simulink model "BrowarModel"  (R2024a)
settings: Solver=ode5  StartTime=0.0  StopTime=inf  FixedStep=0.1  RelTol=1e-3
undefined symbols (not defined in the file or in its folder): localhost, Matrikon, OI
libraries: opclib x24
(part 3 of 9)

== system BrowarModel/Kadz zacierna/FT201 ==
  note: Przetwornik pomiarowy
  In : Inport
  F_gain : Gain  Gain=0
  F_offset : Constant  Value=0
  GUIMon : Gain
  Kompensacja : Constant  Value=Kompensacja
  Product : Product  RndMeth=Zero
  Saturation : Saturate  UpperLimit=100  LowerLimit=0
  Skalowanie (0-100%) : Gain  Gain=100/SrcZakres
  Sum{,1..3} (4 alike) : Sum  Inputs=|++
  Transfer Fcn : TransferFcn  Denominator=[0.3 1]
  Zaklocenia pomiarowe : Subsystem
  Zakres : Constant  Value=Zakres/100
  Out : Outport
  wires:
  Transfer Fcn/1 -> Saturation/1
  F_offset/1 -> Sum3/2
  F_gain/1 -> Sum2/2
  Product/1 -> Sum/1
  Zakres/1 -> Product/2
  Kompensacja/1 -> Sum/2
  Sum/1 -> GUIMon/1
  Skalowanie (0-100%)/1 -> Sum1/1
  Zaklocenia pomiarowe/1(Out) -> Sum1/2
  Sum1/1 -> F_gain/1, Sum2/1
  Sum3/1 -> Transfer Fcn/1
  Sum2/1 -> Sum3/1
  In/1 -> Skalowanie (0-100%)/1
  GUIMon/1 -> Out/1
  Saturation/1 -> Product/1

== system BrowarModel/Kadz zacierna/Kadz zacierna ==
  note: Kadz zacierna
  "Doplyw wody " : Inport
  Doplyw sruty : Inport  Port=2
  Zalaczenie silnika : Inport  Port=3
  "Zadane obroty silnika " : Inport  Port=4
  Sterowanie ogrzewaczem : Inport  Port=5
  Odplyw : Inport  Port=6
  F{211..214,221,231..232,241} (8 alike) : Constant  Value=0
  Kadz zacierna : Subsystem
  Model mieszadla : Subsystem
  Model ogrzewacza : Subsystem
  Silnik elektryczny : Subsystem
  Temperatura sruty : Constant  Value=22
  Temperatura wody : Constant  Value=22
  Terminator1 : Terminator
  Zawor doplywu wody : Subsystem  mask{Fmax=0.2}
      mask prompts: Fmax "Przeplyw maksymalny [m3/s]"
  Poziom : Outport
  Poziom wysoki : Outport  Port=2
  Poziom niski : Outport  Port=3
  Przeplyw wody : Outport  Port=4
  Sensor temperatury gorny : Outport  Port=5
  Sensor temperatury srodkowy : Outport  Port=6
  Sensor temperatury dolny : Outport  Port=7
  Obroty silnika : Outport  Port=8
  Prad silnika : Outport  Port=9
  Silnik Idle : Outport  Port=10
  Silnik Running : Outport  Port=11
  Silnik Alarm : Outport  Port=12
  Jakosc zacieru : Outport  Port=13
  Temperatura : Outport  Port=14
  wires:
  Model mieszadla/1(Obroty zredukowane) -> Kadz zacierna/7(Obroty mieszadla)
  Sterowanie ogrzewaczem/1 -> Model ogrzewacza/1(Sterowanie)
  Doplyw sruty/1 -> Kadz zacierna/3(Doplyw sruty)  "m3/h"
  Kadz zacierna/4(Temperatura sensor gorny) -> Sensor temperatury gorny/1
  Kadz zacierna/5(Temperatura sensor srodkowy) -> Sensor temperatury srodkowy/1
  Kadz zacierna/6(Temperatura sensor dolny) -> Sensor temperatury dolny/1
  Model ogrzewacza/1(Cieplo dostarczone) -> Kadz zacierna/6(Dostepny strumien ciepla)
  Kadz zacierna/1(Poziom) -> Poziom/1, Model mieszadla/1(Poziom)
  Kadz zacierna/2(Poziom wysoki) -> Poziom wysoki/1
  Kadz zacierna/3(Poziom niski) -> Poziom niski/1
  Odplyw/1 -> Kadz zacierna/5(Odplyw)  "m3/s"
  Temperatura wody/1 -> Kadz zacierna/2(Temperatura doplywu wody)
  Temperatura sruty/1 -> Kadz zacierna/4(Temperatura doplywu sruty)
  F221/1 -> Kadz zacierna/8(Wyciek)
  Zalaczenie silnika/1 -> Silnik elektryczny/1(Zalaczenie)
  "Zadane obroty silnika "/1 -> Silnik elektryczny/2(Zadane obroty)
  F232/1 -> Silnik elektryczny/4(Uszkodzenie)
  Model mieszadla/2(Obciazenie) -> Silnik elektryczny/3(Obciazenie zew)
  F231/1 -> Model mieszadla/3(Poslizg przekladni)
  Kadz zacierna/8(Jakosc zacieru) -> Jakosc zacieru/1
  F211/1 -> Zawor doplywu wody/2(Dlawienie)
  "Doplyw wody "/1 -> Zawor doplywu wody/1(Sterowanie)
  F212/1 -> Zawor doplywu wody/3(Przeciek)
  F213/1 -> Zawor doplywu wody/4(Wyciek)
  F214/1 -> Zawor doplywu wody/5(Brak)
  Zawor doplywu wody/1(Przeplyw) -> Przeplyw wody/1, Kadz zacierna/1(Doplyw wody)
  Silnik elektryczny/1(Obroty) -> Model mieszadla/2(Obroty), Obroty silnika/1
  Silnik elektryczny/2(Prad) -> Prad silnika/1
  Silnik elektryczny/3(Idle) -> Silnik Idle/1
  Silnik elektryczny/4(Running) -> Silnik Running/1
  Silnik elektryczny/5(Alarm) -> Silnik Alarm/1
  Kadz zacierna/7(Temperatura dna) -> Terminator1/1
  F241/1 -> Model ogrzewacza/2(Spadek mocy)
  Kadz zacierna/9(Temperatura srednia) -> Temperatura/1

== system BrowarModel/Kadz zacierna/LT202 ==
  note: Przetwornik pomiarowy
  In : Inport
  F_gain : Gain  Gain=0
  F_offset : Constant  Value=0
  GUIMon : Gain
  Kompensacja : Constant  Value=Kompensacja
  Product : Product  RndMeth=Zero
  Saturation : Saturate  UpperLimit=100  LowerLimit=0
  Skalowanie (0-100%) : Gain  Gain=100/SrcZakres
  Sum{,1..3} (4 alike) : Sum  Inputs=|++
  Transfer Fcn : TransferFcn  Denominator=[0.3 1]
  Zaklocenia pomiarowe : Subsystem
  Zakres : Constant  Value=Zakres/100
  Out : Outport
  wires:
  Saturation/1 -> Product/1
  GUIMon/1 -> Out/1
  In/1 -> Skalowanie (0-100%)/1
  Sum2/1 -> Sum3/1
  Sum3/1 -> Transfer Fcn/1
  Sum1/1 -> Sum2/1, F_gain/1
  Zaklocenia pomiarowe/1(Out) -> Sum1/2
  Skalowanie (0-100%)/1 -> Sum1/1
  Sum/1 -> GUIMon/1
  Kompensacja/1 -> Sum/2
  Zakres/1 -> Product/2
  Product/1 -> Sum/1
  F_gain/1 -> Sum2/2
  F_offset/1 -> Sum3/2
  Transfer Fcn/1 -> Saturation/1

== system BrowarModel/Kadz zacierna/LT202H ==
  note: Przetwornik pomiarowy
  In : Inport
  FT : Constant  Value=0
  FT_value : Constant  Value=0
  GUIMon : Gain
  Switch : Switch  Threshold=0.5  SaturateOnIntegerOverflow=off  InputSameDT=off
  Out : Outport
  wires:
  In/1 -> Switch/3
  GUIMon/1 -> Out/1
  FT/1 -> Switch/2
  Switch/1 -> GUIMon/1
  FT_value/1 -> Switch/1

== system BrowarModel/Kadz zacierna/LT202L ==
  note: Przetwornik pomiarowy
  In : Inport
  FT : Constant  Value=0
  FT_value : Constant  Value=0
  GUIMon : Gain
  Switch : Switch  Threshold=0.5  SaturateOnIntegerOverflow=off  InputSameDT=off
  Out : Outport
  wires:
  FT_value/1 -> Switch/1
  Switch/1 -> GUIMon/1
  FT/1 -> Switch/2
  GUIMon/1 -> Out/1
  In/1 -> Switch/3

== system BrowarModel/Kadz zacierna/LV201 ==
  note: Sterowanie
  GUIMon : Gain
  Lokalne : Constant  Value=0
  Wybor : Switch  Threshold=0.5  SaturateOnIntegerOverflow=off  InputSameDT=off
  Out : Outport
  wires:
  GUIMon/1 -> Out/1
  Wybor/1 -> GUIMon/1
  [TrybSter] -> Wybor/2
  [LV201] -> Wybor/1
  Lokalne/1 -> Wybor/3

== system BrowarModel/Kadz zacierna/QT204 ==
  note: Przetwornik pomiarowy
  In : Inport
  FT : Constant  Value=0
  FT_value : Constant  Value=0
  GUIMon : Gain
  Granica : Constant  Value=0.8
  Saturation : Saturate  UpperLimit=1  LowerLimit=0
  Saturation1 : Saturate  UpperLimit=1  LowerLimit=0
  Sensor max : RelationalOperator  InputSameDT=off
  Sum5 : Sum  Inputs=|++
  Switch : Switch  Threshold=0.5  SaturateOnIntegerOverflow=off  InputSameDT=off
  Zaklocenia : Subsystem
  Out : Outport
  wires:
  FT_value/1 -> Switch/1
  Switch/1 -> GUIMon/1
  FT/1 -> Switch/2
  GUIMon/1 -> Out/1
  In/1 -> Saturation/1
  Saturation1/1 -> Switch/3
  Saturation/1 -> Sum5/1, Zaklocenia/1(In)
  Sum5/1 -> Sensor max/1
  Zaklocenia/1(Out) -> Sum5/2
  Granica/1 -> Sensor max/2
  Sensor max/1 -> Saturation1/1

== system BrowarModel/Kadz zacierna/ST205 ==
  note: Przetwornik pomiarowy
  In : Inport
  F_gain : Gain  Gain=0
  F_offset : Constant  Value=0
  GUIMon : Gain
  Kompensacja : Constant  Value=Kompensacja
  Product : Product  RndMeth=Zero
  Saturation : Saturate  UpperLimit=100  LowerLimit=0
  Skalowanie (0-100%) : Gain  Gain=100/SrcZakres
  Sum{,1..3} (4 alike) : Sum  Inputs=|++
  Transfer Fcn : TransferFcn  Denominator=[0.3 1]
  Zaklocenia pomiarowe : Subsystem
  Zakres : Constant  Value=Zakres/100
  Out : Outport
  wires:
  Saturation/1 -> Product/1
  GUIMon/1 -> Out/1
  In/1 -> Skalowanie (0-100%)/1
  Sum2/1 -> Sum3/1
  Sum3/1 -> Transfer Fcn/1
  Sum1/1 -> Sum2/1, F_gain/1
  Zaklocenia pomiarowe/1(Out) -> Sum1/2
  Skalowanie (0-100%)/1 -> Sum1/1
  Sum/1 -> GUIMon/1
  Kompensacja/1 -> Sum/2
  Zakres/1 -> Product/2
  Product/1 -> Sum/1
  F_gain/1 -> Sum2/2
  F_offset/1 -> Sum3/2
  Transfer Fcn/1 -> Saturation/1

== system BrowarModel/Kadz zacierna/TT203H ==
  note: Przetwornik pomiarowy
  In : Inport
  F_gain : Gain  Gain=0
  F_offset : Constant  Value=0
  GUIMon : Gain
  Kompensacja : Constant  Value=Kompensacja
  Product : Product  RndMeth=Zero
  Saturation : Saturate  UpperLimit=100  LowerLimit=0
  Skalowanie (0-100%) : Gain  Gain=100/SrcZakres
  Sum{,1..3} (4 alike) : Sum  Inputs=|++
  Transfer Fcn : TransferFcn  Denominator=[0.3 1]
  Zaklocenia pomiarowe : Subsystem
  Zakres : Constant  Value=Zakres/100
  Out : Outport
  wires:
  Transfer Fcn/1 -> Saturation/1
  F_offset/1 -> Sum3/2
  F_gain/1 -> Sum2/2
  Product/1 -> Sum/1
  Zakres/1 -> Product/2
  Kompensacja/1 -> Sum/2
  Sum/1 -> GUIMon/1
  Skalowanie (0-100%)/1 -> Sum1/1
  Zaklocenia pomiarowe/1(Out) -> Sum1/2
  Sum1/1 -> F_gain/1, Sum2/1
  Sum3/1 -> Transfer Fcn/1
  Sum2/1 -> Sum3/1
  In/1 -> Skalowanie (0-100%)/1
  GUIMon/1 -> Out/1
  Saturation/1 -> Product/1

== system BrowarModel/Kadz zacierna/TT203L ==
  note: Przetwornik pomiarowy
  In : Inport
  F_gain : Gain  Gain=0
  F_offset : Constant  Value=0
  GUIMon : Gain
  Kompensacja : Constant  Value=Kompensacja
  Product : Product  RndMeth=Zero
  Saturation : Saturate  UpperLimit=100  LowerLimit=0
  Skalowanie (0-100%) : Gain  Gain=100/SrcZakres
  Sum{,1..3} (4 alike) : Sum  Inputs=|++
  Transfer Fcn : TransferFcn  Denominator=[0.3 1]
  Zaklocenia pomiarowe : Subsystem
  Zakres : Constant  Value=Zakres/100
  Out : Outport
  wires:
  Transfer Fcn/1 -> Saturation/1
  F_offset/1 -> Sum3/2
  F_gain/1 -> Sum2/2
  Product/1 -> Sum/1
  Zakres/1 -> Product/2
  Kompensacja/1 -> Sum/2
  Sum/1 -> GUIMon/1
  Skalowanie (0-100%)/1 -> Sum1/1
  Zaklocenia pomiarowe/1(Out) -> Sum1/2
  Sum1/1 -> F_gain/1, Sum2/1
  Sum3/1 -> Transfer Fcn/1
  Sum2/1 -> Sum3/1
  In/1 -> Skalowanie (0-100%)/1
  GUIMon/1 -> Out/1
  Saturation/1 -> Product/1

== system BrowarModel/Kadz zacierna/TT203M ==
  note: Przetwornik pomiarowy
  In : Inport
  F_gain : Gain  Gain=0
  F_offset : Constant  Value=0
  GUIMon : Gain
  Kompensacja : Constant  Value=Kompensacja
  Product : Product  RndMeth=Zero
  Saturation : Saturate  UpperLimit=100  LowerLimit=0
  Skalowanie (0-100%) : Gain  Gain=100/SrcZakres
  Sum{,1..3} (4 alike) : Sum  Inputs=|++
  Transfer Fcn : TransferFcn  Denominator=[0.3 1]
  Zaklocenia pomiarowe : Subsystem
  Zakres : Constant  Value=Zakres/100
  Out : Outport
  wires:
  Saturation/1 -> Product/1
  GUIMon/1 -> Out/1
  In/1 -> Skalowanie (0-100%)/1
  Sum2/1 -> Sum3/1
  Sum3/1 -> Transfer Fcn/1
  Sum1/1 -> Sum2/1, F_gain/1
  Zaklocenia pomiarowe/1(Out) -> Sum1/2
  Skalowanie (0-100%)/1 -> Sum1/1
  Sum/1 -> GUIMon/1
  Kompensacja/1 -> Sum/2
  Zakres/1 -> Product/2
  Product/1 -> Sum/1
  F_gain/1 -> Sum2/2
  F_offset/1 -> Sum3/2
  Transfer Fcn/1 -> Saturation/1

== system BrowarModel/Kadz zacierna/TV203 ==
  note: Sterowanie
  GUIMon : Gain
  Lokalne : Constant  Value=0
  Wybor : Switch  Threshold=0.5  SaturateOnIntegerOverflow=off  InputSameDT=off
  Out : Outport
  wires:
  Lokalne/1 -> Wybor/3
  [TV203] -> Wybor/1
  [TrybSter] -> Wybor/2
  Wybor/1 -> GUIMon/1
  GUIMon/1 -> Out/1

== system BrowarModel/Kadz zacierna/XV205 ==
  note: Sterowanie
  GUIMon : Gain
  Lokalne : Constant  Value=0
  Wybor : Switch  Threshold=0.5  SaturateOnIntegerOverflow=off  InputSameDT=off
  Out : Outport
  wires:
  Lokalne/1 -> Wybor/3
  [XV205] -> Wybor/1
  [TrybSter] -> Wybor/2
  Wybor/1 -> GUIMon/1
  GUIMon/1 -> Out/1

== system BrowarModel/Kadz zacierna/XV205SP ==
  note: Sterowanie
  GUIMon : Gain
  Lokalne : Constant  Value=100
  Wybor : Switch  Threshold=0.5  SaturateOnIntegerOverflow=off  InputSameDT=off
  Out : Outport
  wires:
  Lokalne/1 -> Wybor/3
  [XV205SP] -> Wybor/1
  [TrybSter] -> Wybor/2
  Wybor/1 -> GUIMon/1
  GUIMon/1 -> Out/1

== system BrowarModel/Mlyn browarniany/ET103 ==
  note: Przetwornik pomiarowy
  In : Inport
  F_gain : Gain  Gain=0
  F_offset : Constant  Value=0
  GUIMon : Gain
  Kompensacja : Constant  Value=Kompensacja
  Product : Product  RndMeth=Zero
  Saturation : Saturate  UpperLimit=100  LowerLimit=0
  Skalowanie (0-100%) : Gain  Gain=100/SrcZakres
  Sum{,1..3} (4 alike) : Sum  Inputs=|++
  Transfer Fcn : TransferFcn  Denominator=[0.3 1]
  Zaklocenia pomiarowe : Subsystem
  Zakres : Constant  Value=Zakres/100
  Out : Outport
  wires:
  Transfer Fcn/1 -> Saturation/1
  F_offset/1 -> Sum3/2
  F_gain/1 -> Sum2/2
  Product/1 -> Sum/1
  Zakres/1 -> Product/2
  Kompensacja/1 -> Sum/2
  Sum/1 -> GUIMon/1
  Skalowanie (0-100%)/1 -> Sum1/1
  Zaklocenia pomiarowe/1(Out) -> Sum1/2
  Sum1/1 -> F_gain/1, Sum2/1
  Sum3/1 -> Transfer Fcn/1
  Sum2/1 -> Sum3/1
  In/1 -> Skalowanie (0-100%)/1
  GUIMon/1 -> Out/1
  Saturation/1 -> Product/1

== system BrowarModel/Mlyn browarniany/ET105 ==
  note: Przetwornik pomiarowy
  In : Inport
  F_gain : Gain  Gain=0
  F_offset : Constant  Value=0
  GUIMon : Gain
  Kompensacja : Constant  Value=Kompensacja
  Product : Product  RndMeth=Zero
  Saturation : Saturate  UpperLimit=100  LowerLimit=0
  Skalowanie (0-100%) : Gain  Gain=100/SrcZakres
  Sum{,1..3} (4 alike) : Sum  Inputs=|++
  Transfer Fcn : TransferFcn  Denominator=[0.3 1]
  Zaklocenia pomiarowe : Subsystem
  Zakres : Constant  Value=Zakres/100
  Out : Outport
  wires:
  Saturation/1 -> Product/1
  GUIMon/1 -> Out/1
  In/1 -> Skalowanie (0-100%)/1
  Sum2/1 -> Sum3/1
  Sum3/1 -> Transfer Fcn/1
  Sum1/1 -> Sum2/1, F_gain/1
  Zaklocenia pomiarowe/1(Out) -> Sum1/2
  Skalowanie (0-100%)/1 -> Sum1/1
  Sum/1 -> GUIMon/1
  Kompensacja/1 -> Sum/2
  Zakres/1 -> Product/2
  Product/1 -> Sum/1
  F_gain/1 -> Sum2/2
  F_offset/1 -> Sum3/2
  Transfer Fcn/1 -> Saturation/1

== system BrowarModel/Mlyn browarniany/FT105 ==
  note: Przetwornik pomiarowy
  In : Inport
  F_gain : Gain  Gain=0
  F_offset : Constant  Value=0
  GUIMon : Gain
  Kompensacja : Constant  Value=Kompensacja
  Product : Product  RndMeth=Zero
  Saturation : Saturate  UpperLimit=100  LowerLimit=0
  Skalowanie (0-100%) : Gain  Gain=100/SrcZakres
  Sum{,1..3} (4 alike) : Sum  Inputs=|++
  Transfer Fcn : TransferFcn  Denominator=[0.3 1]
  Zaklocenia pomiarowe : Subsystem
  Zakres : Constant  Value=Zakres/100
  Out : Outport
  wires:
  Saturation/1 -> Product/1
  GUIMon/1 -> Out/1
  In/1 -> Skalowanie (0-100%)/1
  Sum2/1 -> Sum3/1
  Sum3/1 -> Transfer Fcn/1
  Sum1/1 -> Sum2/1, F_gain/1
  Zaklocenia pomiarowe/1(Out) -> Sum1/2
  Skalowanie (0-100%)/1 -> Sum1/1
  Sum/1 -> GUIMon/1
  Kompensacja/1 -> Sum/2
  Zakres/1 -> Product/2
  Product/1 -> Sum/1
  F_gain/1 -> Sum2/2
  F_offset/1 -> Sum3/2
  Transfer Fcn/1 -> Saturation/1

== system BrowarModel/Mlyn browarniany/FV103 ==
  note: Sterowanie
  GUIMon : Gain
  Lokalne : Constant  Value=0
  Wybor : Switch  Threshold=0.5  SaturateOnIntegerOverflow=off  InputSameDT=off
  Out : Outport
  wires:
  Lokalne/1 -> Wybor/3
  [FV103] -> Wybor/1
  [TrybSter] -> Wybor/2
  Wybor/1 -> GUIMon/1
  GUIMon/1 -> Out/1

== system BrowarModel/Mlyn browarniany/FV103SP ==
  note: Sterowanie
  GUIMon : Gain
  Lokalne : Constant  Value=65.3333
  Wybor : Switch  Threshold=0.5  SaturateOnIntegerOverflow=off  InputSameDT=off
  Out : Outport
  wires:
  GUIMon/1 -> Out/1
  Wybor/1 -> GUIMon/1
  [TrybSter] -> Wybor/2
  [FV103SP] -> Wybor/1
  Lokalne/1 -> Wybor/3

== system BrowarModel/Mlyn browarniany/FV105 ==
  note: Sterowanie
  GUIMon : Gain
  Lokalne : Constant  Value=0
  Wybor : Switch  Threshold=0.5  SaturateOnIntegerOverflow=off  InputSameDT=off
  Out : Outport
  wires:
  Lokalne/1 -> Wybor/3
  [FV105] -> Wybor/1
  [TrybSter] -> Wybor/2
  Wybor/1 -> GUIMon/1
  GUIMon/1 -> Out/1

== system BrowarModel/Mlyn browarniany/FV105SP ==
  note: Sterowanie
  GUIMon : Gain
  Lokalne : Constant  Value=100
  Wybor : Switch  Threshold=0.5  SaturateOnIntegerOverflow=off  InputSameDT=off
  Out : Outport
  wires:
  Lokalne/1 -> Wybor/3
  [FV105SP] -> Wybor/1
  [TrybSter] -> Wybor/2
  Wybor/1 -> GUIMon/1
  GUIMon/1 -> Out/1

== system BrowarModel/Mlyn browarniany/LT102 ==
  note: Przetwornik pomiarowy
  In : Inport
  F_gain : Gain  Gain=0
  F_offset : Constant  Value=0
  GUIMon : Gain
  Kompensacja : Constant  Value=Kompensacja
  Product : Product  RndMeth=Zero
  Saturation : Saturate  UpperLimit=100  LowerLimit=0
  Skalowanie (0-100%) : Gain  Gain=100/SrcZakres
  Sum{,1..3} (4 alike) : Sum  Inputs=|++
  Transfer Fcn : TransferFcn  Denominator=[0.3 1]
  Zaklocenia pomiarowe : Subsystem
  Zakres : Constant  Value=Zakres/100
  Out : Outport
  wires:
  Saturation/1 -> Product/1
  GUIMon/1 -> Out/1
  In/1 -> Skalowanie (0-100%)/1
  Sum2/1 -> Sum3/1
  Sum3/1 -> Transfer Fcn/1
  Sum1/1 -> Sum2/1, F_gain/1
  Zaklocenia pomiarowe/1(Out) -> Sum1/2
  Skalowanie (0-100%)/1 -> Sum1/1
  Sum/1 -> GUIMon/1
  Kompensacja/1 -> Sum/2
  Zakres/1 -> Product/2
  Product/1 -> Sum/1
  F_gain/1 -> Sum2/2
  F_offset/1 -> Sum3/2
  Transfer Fcn/1 -> Saturation/1

== system BrowarModel/Mlyn browarniany/LT102H ==
  note: Przetwornik pomiarowy
  In : Inport
  FT : Constant  Value=0
  FT_value : Constant  Value=0
  GUIMon : Gain
  Switch : Switch  Threshold=0.5  SaturateOnIntegerOverflow=off  InputSameDT=off
  Out : Outport
  wires:
  In/1 -> Switch/3
  GUIMon/1 -> Out/1
  FT/1 -> Switch/2
  Switch/1 -> GUIMon/1
  FT_value/1 -> Switch/1

== system BrowarModel/Mlyn browarniany/LT102L ==
  note: Przetwornik pomiarowy
  In : Inport
  FT : Constant  Value=0
  FT_value : Constant  Value=0
  GUIMon : Gain
  Switch : Switch  Threshold=0.5  SaturateOnIntegerOverflow=off  InputSameDT=off
  Out : Outport
  wires:
  FT_value/1 -> Switch/1
  Switch/1 -> GUIMon/1
  FT/1 -> Switch/2
  GUIMon/1 -> Out/1
  In/1 -> Switch/3

== system BrowarModel/Mlyn browarniany/LT104H ==
  note: Przetwornik pomiarowy
  In : Inport
  FT : Constant  Value=0
  FT_value : Constant  Value=0
  GUIMon : Gain
  Switch : Switch  Threshold=0.5  SaturateOnIntegerOverflow=off  InputSameDT=off
  Out : Outport
  wires:
  FT_value/1 -> Switch/1
  Switch/1 -> GUIMon/1
  FT/1 -> Switch/2
  GUIMon/1 -> Out/1
  In/1 -> Switch/3

== system BrowarModel/Mlyn browarniany/LT104L ==
  note: Przetwornik pomiarowy
  In : Inport
  FT : Constant  Value=0
  FT_value : Constant  Value=0
  GUIMon : Gain
  Switch : Switch  Threshold=0.5  SaturateOnIntegerOverflow=off  InputSameDT=off
  Out : Outport
  wires:
  In/1 -> Switch/3
  GUIMon/1 -> Out/1
  FT/1 -> Switch/2
  Switch/1 -> GUIMon/1
  FT_value/1 -> Switch/1

== system BrowarModel/Mlyn browarniany/LV101 ==
  note: Sterowanie
  GUIMon : Gain
  Lokalne : Constant  Value=0
  Wybor : Switch  Threshold=0.5  SaturateOnIntegerOverflow=off  InputSameDT=off
  Out : Outport
  wires:
  GUIMon/1 -> Out/1
  Wybor/1 -> GUIMon/1
  [TrybSter] -> Wybor/2
  [LV101] -> Wybor/1
  Lokalne/1 -> Wybor/3

== system BrowarModel/Mlyn browarniany/Mlyn browarniany ==
  note: Mlyn browarniany
  Doplyw zasobnika : Inport
  Zalaczenie silnika dozownika : Inport  Port=2
  Zadane obroty silnika dozownika : Inport  Port=3
  Zalaczenie silnika walcow : Inport  Port=4
  Zadane obroty silnika walcow : Inport  Port=5
  Dozownik mlyna : Subsystem
  F{111..114,121,131..136,141..146} (17 alike) : Constant  Value=0
  Walce mlyna : Subsystem
  Zasobnik dozownika slodu : Subsystem
  Zawor doplywu slodu : Subsystem  mask{Fmax=0.2}
      mask prompts: Fmax "Przeplyw maksymalny [m3/s]"
  Przeplyw : Outport
  Poziom zasobnika : Outport  Port=2
  Poziom wysoki zasobnika : Outport  Port=3
  Poziom niski zasobnika : Outport  Port=4
  Obroty silnika dozownika : Outport  Port=5
  Prad silnika dozownika : Outport  Port=6
  Silnik dozownika Idle : Outport  Port=7
  Silnik dozownika Running : Outport  Port=8
  Silnik dozownika Alarm : Outport  Port=9
  Temperatura lozyska dozownika : Outport  Port=10
  Poziom wysoki komory : Outport  Port=11
  Poziom niski komory : Outport  Port=12
  Obroty silnika walcow : Outport  Port=13
  Prad silnika walcow : Outport  Port=14
  Silnik walcow Idle : Outport  Port=15
  Silnik walcow Running : Outport  Port=16
  Silnik walcow Alarm : Outport  Port=17
  Temperatura lozyska walcow : Outport  Port=18
  wires:
  Zasobnik dozownika slodu/1(Poziom) -> Dozownik mlyna/3(Poziom zasobnika), Poziom zasobnika/1
  Dozownik mlyna/1(Przeplyw) -> Walce mlyna/3(Doplyw do komory), Zasobnik dozownika slodu/2(Odplyw)
  Zalaczenie silnika dozownika/1 -> Dozownik mlyna/1(Zalaczenie silnika)
  Walce mlyna/2(Wypelnienie) -> Dozownik mlyna/4(Wyplnienie komory)
  Walce mlyna/1(Przeplyw) -> Przeplyw/1
  Zasobnik dozownika slodu/2(Poziom HI) -> Poziom wysoki zasobnika/1
  Zasobnik dozownika slodu/3(Poziom LO) -> Poziom niski zasobnika/1
  F121/1 -> Zasobnik dozownika slodu/3(Wyciek)
  F111/1 -> Zawor doplywu slodu/2(Dlawienie)
  Zawor doplywu slodu/1(Przeplyw) -> Zasobnik dozownika slodu/1(Doplyw)
  Doplyw zasobnika/1 -> Zawor doplywu slodu/1(Sterowanie)
  F131/1 -> Dozownik mlyna/5(Zanieczyszczenie lopatek)
  Dozownik mlyna/2(Temperatura lozyska) -> Temperatura lozyska dozownika/1
  Dozownik mlyna/4(Prad silnika) -> Prad silnika dozownika/1
  Dozownik mlyna/3(Obroty silnika) -> Obroty silnika dozownika/1
  Zadane obroty silnika dozownika/1 -> Dozownik mlyna/2("Zadane obroty silnika ")
  F136/1 -> Dozownik mlyna/10(Uszkodzenie silnika)
  Zalaczenie silnika walcow/1 -> Walce mlyna/1(Zalaczenie silnika)
  Zadane obroty silnika walcow/1 -> Walce mlyna/2("Zadane obroty silnika ")
  F146/1 -> Walce mlyna/9(Uszkodzenie silnika)
  Walce mlyna/8(Komora nad walcami poziom HI) -> Poziom wysoki komory/1
  Walce mlyna/9(Komora nad walcami poziom LO) -> Poziom niski komory/1
  Walce mlyna/4(Prad silnika) -> Prad silnika walcow/1
  Walce mlyna/3(Obroty silnika) -> Obroty silnika walcow/1
  F141/1 -> Walce mlyna/4(Zanieczyszczenie walcow)
  F142/1 -> Walce mlyna/5(Blokada przeplywu)
  F144/1 -> Walce mlyna/7(Poslizg przekladni)
  F145/1 -> Walce mlyna/8(Uszkodzenie lozyska)
  Walce mlyna/10(Temperatura lozyska) -> Temperatura lozyska walcow/1
  F112/1 -> Zawor doplywu slodu/3(Przeciek)
  F113/1 -> Zawor doplywu slodu/4(Wyciek)
  F114/1 -> Zawor doplywu slodu/5(Brak)
  Dozownik mlyna/5(Silnik Idle) -> Silnik dozownika Idle/1
  Dozownik mlyna/6(Silnik Running) -> Silnik dozownika Running/1
  Dozownik mlyna/7(Silnik Alarm) -> Silnik dozownika Alarm/1
  Walce mlyna/5(Silnik Idle) -> Silnik walcow Idle/1
  Walce mlyna/6(Silnik Running) -> Silnik walcow Running/1
  Walce mlyna/7(Silnik Alarm) -> Silnik walcow Alarm/1
  F132/1 -> Dozownik mlyna/6(Blokada przeplywu)
  F135/1 -> Dozownik mlyna/9(Uszkodzenie lozyska)
  F134/1 -> Dozownik mlyna/8("Poslizg przekladni ")
  F133/1 -> Dozownik mlyna/7(Przeciek w dozowniku)
  F143/1 -> Walce mlyna/6(Przeciek materialu przez walce)

== system BrowarModel/Mlyn browarniany/ST103 ==
  note: Przetwornik pomiarowy
  In : Inport
  F_gain : Gain  Gain=0
  F_offset : Constant  Value=0
  GUIMon : Gain
  Kompensacja : Constant  Value=Kompensacja
  Product : Product  RndMeth=Zero
  Saturation : Saturate  UpperLimit=100  LowerLimit=0
  Skalowanie (0-100%) : Gain  Gain=100/SrcZakres
  Sum{,1..3} (4 alike) : Sum  Inputs=|++
  Transfer Fcn : TransferFcn  Denominator=[0.3 1]
  Zaklocenia pomiarowe : Subsystem
  Zakres : Constant  Value=Zakres/100
  Out : Outport
  wires:
  Transfer Fcn/1 -> Saturation/1
  F_offset/1 -> Sum3/2
  F_gain/1 -> Sum2/2
  Product/1 -> Sum/1
  Zakres/1 -> Product/2
  Kompensacja/1 -> Sum/2
  Sum/1 -> GUIMon/1
  Skalowanie (0-100%)/1 -> Sum1/1
  Zaklocenia pomiarowe/1(Out) -> Sum1/2
  Sum1/1 -> F_gain/1, Sum2/1
  Sum3/1 -> Transfer Fcn/1
  Sum2/1 -> Sum3/1
  In/1 -> Skalowanie (0-100%)/1
  GUIMon/1 -> Out/1
  Saturation/1 -> Product/1

== system BrowarModel/Mlyn browarniany/ST105 ==
  note: Przetwornik pomiarowy
  In : Inport
  F_gain : Gain  Gain=0
  F_offset : Constant  Value=0
  GUIMon : Gain
  Kompensacja : Constant  Value=Kompensacja
  Product : Product  RndMeth=Zero
  Saturation : Saturate  UpperLimit=100  LowerLimit=0
  Skalowanie (0-100%) : Gain  Gain=100/SrcZakres
  Sum{,1..3} (4 alike) : Sum  Inputs=|++
  Transfer Fcn : TransferFcn  Denominator=[0.3 1]
  Zaklocenia pomiarowe : Subsystem
  Zakres : Constant  Value=Zakres/100
  Out : Outport
  wires:
  Saturation/1 -> Product/1
  GUIMon/1 -> Out/1
  In/1 -> Skalowanie (0-100%)/1
  Sum2/1 -> Sum3/1
  Sum3/1 -> Transfer Fcn/1
  Sum1/1 -> Sum2/1, F_gain/1
  Zaklocenia pomiarowe/1(Out) -> Sum1/2
  Skalowanie (0-100%)/1 -> Sum1/1
  Sum/1 -> GUIMon/1
  Kompensacja/1 -> Sum/2
  Zakres/1 -> Product/2
  Product/1 -> Sum/1
  F_gain/1 -> Sum2/2
  F_offset/1 -> Sum3/2
  Transfer Fcn/1 -> Saturation/1

== system BrowarModel/Mlyn browarniany/TT103 ==
  note: Przetwornik pomiarowy
  In : Inport
  F_gain : Gain  Gain=0
  F_offset : Constant  Value=0
  GUIMon : Gain
  Kompensacja : Constant  Value=Kompensacja
  Product : Product  RndMeth=Zero
  Saturation : Saturate  UpperLimit=100  LowerLimit=0
  Skalowanie (0-100%) : Gain  Gain=100/SrcZakres
  Sum{,1..3} (4 alike) : Sum  Inputs=|++
  Transfer Fcn : TransferFcn  Denominator=[0.3 1]
  Zaklocenia pomiarowe : Subsystem
  Zakres : Constant  Value=Zakres/100
  Out : Outport
  wires:
  Transfer Fcn/1 -> Saturation/1
  F_offset/1 -> Sum3/2
  F_gain/1 -> Sum2/2
  Product/1 -> Sum/1
  Zakres/1 -> Product/2
  Kompensacja/1 -> Sum/2
  Sum/1 -> GUIMon/1
  Skalowanie (0-100%)/1 -> Sum1/1
  Zaklocenia pomiarowe/1(Out) -> Sum1/2
  Sum1/1 -> F_gain/1, Sum2/1
  Sum3/1 -> Transfer Fcn/1
  Sum2/1 -> Sum3/1
  In/1 -> Skalowanie (0-100%)/1
  GUIMon/1 -> Out/1
  Saturation/1 -> Product/1

== system BrowarModel/Mlyn browarniany/TT105 ==
  note: Przetwornik pomiarowy
  In : Inport
  F_gain : Gain  Gain=0
  F_offset : Constant  Value=0
  GUIMon : Gain
  Kompensacja : Constant  Value=Kompensacja
  Product : Product  RndMeth=Zero
  Saturation : Saturate  UpperLimit=100  LowerLimit=0
  Skalowanie (0-100%) : Gain  Gain=100/SrcZakres
  Sum{,1..3} (4 alike) : Sum  Inputs=|++
  Transfer Fcn : TransferFcn  Denominator=[0.3 1]
  Zaklocenia pomiarowe : Subsystem
  Zakres : Constant  Value=Zakres/100
  Out : Outport
  wires:
  Saturation/1 -> Product/1
  GUIMon/1 -> Out/1
  In/1 -> Skalowanie (0-100%)/1
  Sum2/1 -> Sum3/1
  Sum3/1 -> Transfer Fcn/1
  Sum1/1 -> Sum2/1, F_gain/1
  Zaklocenia pomiarowe/1(Out) -> Sum1/2
  Skalowanie (0-100%)/1 -> Sum1/1
  Sum/1 -> GUIMon/1
  Kompensacja/1 -> Sum/2
  Zakres/1 -> Product/2
  Product/1 -> Sum/1
  F_gain/1 -> Sum2/2
  F_offset/1 -> Sum3/2
  Transfer Fcn/1 -> Saturation/1

== system BrowarModel/Schladzacz/Schladzacz ==
  note: Schladzacz
  Temperatura we : Inport
  Przeplyw we : Inport  Port=2
  Sterowanie : Inport  Port=3
  " Stala C->K " : Sum
  "C -> K " : Sum
  C->K : Constant  Value=273.6
  Cieplo wejsciowe brzeczki : Fcn  Expr=u(1)*u(2)*u(3)
  Cieplo wejsciowe wody lodowej : Fcn  Expr=u(1)*u(2)*u(3)
  Cieplo wlasciwe brzeczki : Constant  Value=4189.9
  Cieplo wlasciwe wody : Constant  Value=4189.9
  Cieplo wyjsciowe brzeczki : Sum  Inputs=+-
  Cieplo wyjsciowe wody : Sum
  Gestosc : Gain  Gain=1000
  "K -> C" : Sum  Inputs=+-
  "K -> C " : Sum  Inputs=+-
  Max przeplyw wody lodowej : Constant  Value=5*1000
  Mux : Mux  Inputs=6
  Mux{1..5} (5 alike) : Mux  Inputs=3
  Product : Product  RndMeth=Zero
  Przekazane cieplo : Fcn  Expr=0.90*u(1)*u(2)*u(3)
  Sat (0..100%) : Saturate  UpperLimit=100  LowerLimit=0
  Sat1 : Saturate  UpperLimit=inf  LowerLimit=0.0001
  Sat2 : Saturate  UpperLimit=inf  LowerLimit=0.0001
  Saturation : Saturate  UpperLimit=373.6  LowerLimit=273.6
  Skalowanie : Gain  Gain=1/100
  Spadek temperatury : Sum  Inputs=+-
  Stala C->K : Constant  Value=273.6
  "Stala C->K " : Constant  Value=273.6
  Temperatura wody lodowej : Constant  Value=4
  Temperatura wyjsciowa : Fcn  Expr=(u(1)*u(2)*u(3)+u(4)*u(5)*u(6))/(u(1)*u(2)+u(4)*u(5))
  Temperatura wyjsciowa brzeczki : Fcn  Expr=u(3)/(u(1)*u(2))
  Temperatyra wyjsciowa wody : Fcn  Expr=u(1)/(u(2)*u(3))
  Temperatura wy : Outport
  Przeplyw wy : Outport  Port=2
  Temperatura wody we : Outport  Port=3
  Temperatura wody wy : Outport  Port=4
  wires:
  C->K/1 -> " Stala C->K "/2, "C -> K "/1
  Temperatura wody lodowej/1 -> "C -> K "/2, Temperatura wody we/1
  Temperatura we/1 -> " Stala C->K "/1
  Przeplyw we/1 -> Przeplyw wy/1, Gestosc/1  "m3/s"
  "C -> K "/1 -> Mux/6, Mux4/3
  Cieplo wlasciwe wody/1 -> Mux/2, Mux1/2, Mux2/2, Mux3/2  "J/(kg * deg K)"
  " Stala C->K "/1 -> Mux/3, Spadek temperatury/1, Mux2/3  "deg K"
  Product/1 -> Sat2/1
  Cieplo wlasciwe brzeczki/1 -> Mux/5, Mux4/2, Mux5/2  "J/(kg * deg K)"
  Mux/1 -> Temperatura wyjsciowa/1
  Temperatura wyjsciowa/1 -> Saturation/1
  Saturation/1 -> Spadek temperatury/2  "deg K"
  Spadek temperatury/1 -> Mux1/3
  Mux1/1 -> Przekazane cieplo/1
  Mux2/1 -> Cieplo wejsciowe brzeczki/1
  Cieplo wejsciowe brzeczki/1 -> Cieplo wyjsciowe brzeczki/1
  Przekazane cieplo/1 -> Cieplo wyjsciowe brzeczki/2, Cieplo wyjsciowe wody/1
  Cieplo wyjsciowe brzeczki/1 -> Mux3/3  "J"
  Mux3/1 -> Temperatura wyjsciowa brzeczki/1
  Temperatura wyjsciowa brzeczki/1 -> "K -> C"/1  "deg K"
  Stala C->K/1 -> "K -> C"/2  "deg K"
  Mux4/1 -> Cieplo wejsciowe wody lodowej/1
  Cieplo wejsciowe wody lodowej/1 -> Cieplo wyjsciowe wody/2
  Cieplo wyjsciowe wody/1 -> Mux5/1  "J"
  Mux5/1 -> Temperatyra wyjsciowa wody/1
  Temperatyra wyjsciowa wody/1 -> "K -> C "/1  "deg K"
  "Stala C->K "/1 -> "K -> C "/2  "deg K"
  Gestosc/1 -> Sat1/1  "kg/s"
  Sat (0..100%)/1 -> Skalowanie/1
  Sterowanie/1 -> Sat (0..100%)/1
  Skalowanie/1 -> Product/1
  Max przeplyw wody lodowej/1 -> Product/2  "kg/sek"
  Sat1/1 -> Mux/1, Mux1/1, Mux2/1, Mux3/1
  "K -> C"/1 -> Temperatura wy/1  "deg C"
  Sat2/1 -> Mux/4, Mux4/1, Mux5/3
  "K -> C "/1 -> Temperatura wody wy/1  "deg C"

== system BrowarModel/Schladzacz/TT601 ==
  note: Przetwornik pomiarowy
  In : Inport
  F_gain : Gain  Gain=0
  F_offset : Constant  Value=0
  GUIMon : Gain
  Kompensacja : Constant  Value=Kompensacja
  Product : Product  RndMeth=Zero
  Saturation : Saturate  UpperLimit=100  LowerLimit=0
  Skalowanie (0-100%) : Gain  Gain=100/SrcZakres
  Sum{,1..3} (4 alike) : Sum  Inputs=|++
  Transfer Fcn : TransferFcn  Denominator=[0.3 1]
  Zaklocenia pomiarowe : Subsystem
  Zakres : Constant  Value=Zakres/100
  Out : Outport
  wires:
  Transfer Fcn/1 -> Saturation/1
  F_offset/1 -> Sum3/2
  F_gain/1 -> Sum2/2
  Product/1 -> Sum/1
  Zakres/1 -> Product/2
  Kompensacja/1 -> Sum/2
  Sum/1 -> GUIMon/1
  Skalowanie (0-100%)/1 -> Sum1/1
  Zaklocenia pomiarowe/1(Out) -> Sum1/2
  Sum1/1 -> F_gain/1, Sum2/1
  Sum3/1 -> Transfer Fcn/1
  Sum2/1 -> Sum3/1
  In/1 -> Skalowanie (0-100%)/1
  GUIMon/1 -> Out/1
  Saturation/1 -> Product/1

== system BrowarModel/Schladzacz/TT602 ==
  note: Przetwornik pomiarowy
  In : Inport
  F_gain : Gain  Gain=0
  F_offset : Constant  Value=0
  GUIMon : Gain
  Kompensacja : Constant  Value=Kompensacja
  Product : Product  RndMeth=Zero
  Saturation : Saturate  UpperLimit=100  LowerLimit=0
  Skalowanie (0-100%) : Gain  Gain=100/SrcZakres
  Sum{,1..3} (4 alike) : Sum  Inputs=|++
  Transfer Fcn : TransferFcn  Denominator=[0.3 1]
  Zaklocenia pomiarowe : Subsystem
  Zakres : Constant  Value=Zakres/100
  Out : Outport
  wires:
  Saturation/1 -> Product/1
  GUIMon/1 -> Out/1
  In/1 -> Skalowanie (0-100%)/1
  Sum2/1 -> Sum3/1
  Sum3/1 -> Transfer Fcn/1
  Sum1/1 -> Sum2/1, F_gain/1
  Zaklocenia pomiarowe/1(Out) -> Sum1/2
  Skalowanie (0-100%)/1 -> Sum1/1
  Sum/1 -> GUIMon/1
  Kompensacja/1 -> Sum/2
  Zakres/1 -> Product/2
  Product/1 -> Sum/1
  F_gain/1 -> Sum2/2
  F_offset/1 -> Sum3/2
  Transfer Fcn/1 -> Saturation/1

== system BrowarModel/Schladzacz/TT603 ==
  note: Przetwornik pomiarowy
  In : Inport
  F_gain : Gain  Gain=0
  F_offset : Constant  Value=0
  GUIMon : Gain
  Kompensacja : Constant  Value=Kompensacja
  Product : Product  RndMeth=Zero
  Saturation : Saturate  UpperLimit=100  LowerLimit=0
  Skalowanie (0-100%) : Gain  Gain=100/SrcZakres
  Sum{,1..3} (4 alike) : Sum  Inputs=|++
  Transfer Fcn : TransferFcn  Denominator=[0.3 1]
  Zaklocenia pomiarowe : Subsystem
  Zakres : Constant  Value=Zakres/100
  Out : Outport
  wires:
  Transfer Fcn/1 -> Saturation/1
  F_offset/1 -> Sum3/2
  F_gain/1 -> Sum2/2
  Product/1 -> Sum/1
  Zakres/1 -> Product/2
  Kompensacja/1 -> Sum/2
  Sum/1 -> GUIMon/1
  Skalowanie (0-100%)/1 -> Sum1/1
  Zaklocenia pomiarowe/1(Out) -> Sum1/2
  Sum1/1 -> F_gain/1, Sum2/1
  Sum3/1 -> Transfer Fcn/1
  Sum2/1 -> Sum3/1
  In/1 -> Skalowanie (0-100%)/1
  GUIMon/1 -> Out/1
  Saturation/1 -> Product/1

== system BrowarModel/Schladzacz/TT604 ==
  note: Przetwornik pomiarowy
  In : Inport
  F_gain : Gain  Gain=0
  F_offset : Constant  Value=0
  GUIMon : Gain
  Kompensacja : Constant  Value=Kompensacja
  Product : Product  RndMeth=Zero
  Saturation : Saturate  UpperLimit=100  LowerLimit=0
  Skalowanie (0-100%) : Gain  Gain=100/SrcZakres
  Sum{,1..3} (4 alike) : Sum  Inputs=|++
  Transfer Fcn : TransferFcn  Denominator=[0.3 1]
  Zaklocenia pomiarowe : Subsystem
  Zakres : Constant  Value=Zakres/100
  Out : Outport
  wires:
  Saturation/1 -> Product/1
  GUIMon/1 -> Out/1
  In/1 -> Skalowanie (0-100%)/1
  Sum2/1 -> Sum3/1
  Sum3/1 -> Transfer Fcn/1
  Sum1/1 -> Sum2/1, F_gain/1
  Zaklocenia pomiarowe/1(Out) -> Sum1/2
  Skalowanie (0-100%)/1 -> Sum1/1
  Sum/1 -> GUIMon/1
  Kompensacja/1 -> Sum/2
  Zakres/1 -> Product/2
  Product/1 -> Sum/1
  F_gain/1 -> Sum2/2
  F_offset/1 -> Sum3/2
  Transfer Fcn/1 -> Saturation/1

== system BrowarModel/Schladzacz/TV601 ==
  note: Sterowanie
  GUIMon : Gain
  Lokalne : Constant  Value=0
  Wybor : Switch  Threshold=0.5  SaturateOnIntegerOverflow=off  InputSameDT=off
  Out : Outport
  wires:
  GUIMon/1 -> Out/1
  Wybor/1 -> GUIMon/1
  [TrybSter] -> Wybor/2
  [TV601] -> Wybor/1
  Lokalne/1 -> Wybor/3

== system BrowarModel/System dozowania chmielu/LT502H ==
  note: Przetwornik pomiarowy
  In : Inport
  FT : Constant  Value=0
  FT_value : Constant  Value=0
  GUIMon : Gain
  Switch : Switch  Threshold=0.5  SaturateOnIntegerOverflow=off  InputSameDT=off
  Out : Outport
  wires:
  In/1 -> Switch/3
  GUIMon/1 -> Out/1
  FT/1 -> Switch/2
  Switch/1 -> GUIMon/1
  FT_value/1 -> Switch/1

== system BrowarModel/System dozowania chmielu/LT502L ==
  note: Przetwornik pomiarowy
  In : Inport
  FT : Constant  Value=0
  FT_value : Constant  Value=0
  GUIMon : Gain
  Switch : Switch  Threshold=0.5  SaturateOnIntegerOverflow=off  InputSameDT=off
  Out : Outport
  wires:
  FT_value/1 -> Switch/1
  Switch/1 -> GUIMon/1
  FT/1 -> Switch/2
  GUIMon/1 -> Out/1
  In/1 -> Switch/3

== system BrowarModel/System dozowania chmielu/LV501 ==
  note: Sterowanie
  GUIMon : Gain
  Lokalne : Constant  Value=0
  Wybor : Switch  Threshold=0.5  SaturateOnIntegerOverflow=off  InputSameDT=off
  Out : Outport
  wires:
  GUIMon/1 -> Out/1
  Wybor/1 -> GUIMon/1
  [TrybSter] -> Wybor/2
  [LV501] -> Wybor/1
  Lokalne/1 -> Wybor/3

== system BrowarModel/System dozowania chmielu/PT503 ==
  note: Przetwornik pomiarowy
  In : Inport
  F_gain : Gain  Gain=0
  F_offset : Constant  Value=0
  GUIMon : Gain
  Kompensacja : Constant  Value=Kompensacja
  Product : Product  RndMeth=Zero
  Saturation : Saturate  UpperLimit=100  LowerLimit=0
  Skalowanie (0-100%) : Gain  Gain=100/SrcZakres
  Sum{,1..3} (4 alike) : Sum  Inputs=|++
  Transfer Fcn : TransferFcn  Denominator=[0.3 1]
  Zaklocenia pomiarowe : Subsystem
  Zakres : Constant  Value=Zakres/100
  Out : Outport
  wires:
  Saturation/1 -> Product/1
  GUIMon/1 -> Out/1
  In/1 -> Skalowanie (0-100%)/1
  Sum2/1 -> Sum3/1
  Sum3/1 -> Transfer Fcn/1
  Sum1/1 -> Sum2/1, F_gain/1
  Zaklocenia pomiarowe/1(Out) -> Sum1/2
  Skalowanie (0-100%)/1 -> Sum1/1
  Sum/1 -> GUIMon/1
  Kompensacja/1 -> Sum/2
  Zakres/1 -> Product/2
  Product/1 -> Sum/1
  F_gain/1 -> Sum2/2
  F_offset/1 -> Sum3/2
  Transfer Fcn/1 -> Saturation/1

== system BrowarModel/System dozowania chmielu/PV503 ==
  note: Sterowanie
  GUIMon : Gain
  Lokalne : Constant  Value=0
  Wybor : Switch  Threshold=0.5  SaturateOnIntegerOverflow=off  InputSameDT=off
  Out : Outport
  wires:
  Lokalne/1 -> Wybor/3
  [PV503] -> Wybor/1
  [TrybSter] -> Wybor/2
  Wybor/1 -> GUIMon/1
  GUIMon/1 -> Out/1

== system BrowarModel/System dozowania chmielu/System dozowania chmielu ==
  note: System dozowania chmielu
  Doplyw zasobnika : Inport
  Zalaczenie pompy : Inport  Port=2
  Sterowanie rusztem : Inport  Port=3
  Oproznianie : Inport  Port=4
  F{511..514,521,531..532,541,551} (9 alike) : Constant  Value=0
  Pozycja sensora max : Constant  Value=0.1*0.1
  Ruszt dozujacy : Subsystem
  Sensor max : RelationalOperator  InputSameDT=off
  Silownik hydrauliczny : Subsystem
  Sterownik rusztu : Subsystem
  Waga : Subsystem
  Zasilacz hydrauliczny : Subsystem
  Zasobnik : Subsystem
  Zawor doplywu chmielu : Subsystem  mask{Fmax=0.05}
      mask prompts: Fmax "Przeplyw maksymalny [m3/s]"
  Zawor trojdrozny : Subsystem
  Poziom wysoki zasobnika : Outport
  Poziom niski zasobnika : Outport  Port=2
  Cisnienie pompy : Outport  Port=3
  Masa : Outport  Port=4
  Odplyw chmielu : Outport  Port=5
  Pozycja : Outport  Port=6
  PozycjaDisc : Outport  Port=7
  Waga poz gora : Outport  Port=8
  Waga poz dol : Outport  Port=9
  wires:
  Ruszt dozujacy/1(Przeplyw) -> Waga/1(Doplyw), Zasobnik/2(Odplyw)
  Silownik hydrauliczny/1(Pozycja) -> Sterownik rusztu/1(Pozycja rusztu), Ruszt dozujacy/1(Pozycja), Pozycja/1, Sensor max/1
  Silownik hydrauliczny/2(Przeplyw pobor) -> Zasilacz hydrauliczny/2(Przeplyw_pobor)
  Zawor trojdrozny/1(Przeplyw sterowanie) -> Silownik hydrauliczny/1(Przeplyw zasilanie)
  Zasilacz hydrauliczny/1(Max przeplyw zasilanie) -> Zawor trojdrozny/2(Przeplyw zasilanie)
  Sterownik rusztu/1(Sterowanie zaworem) -> Zawor trojdrozny/1(Sterowanie rusztem)
  Waga/1(Masa) -> Masa/1  "kg"
  Zasobnik/1(Poziom) -> Ruszt dozujacy/2(Poziom_w_zbiorniku)
  Zasobnik/2(Poziom HI) -> Poziom wysoki zasobnika/1
  Zasobnik/3(Poziom LO) -> Poziom niski zasobnika/1
  F521/1 -> Zasobnik/3(Wyciek)
  Zawor doplywu chmielu/1(Przeplyw) -> Zasobnik/1(Doplyw)
  Zasilacz hydrauliczny/2(Cisnienie zasilania) -> Cisnienie pompy/1
  F531/1 -> Zasilacz hydrauliczny/3(Spadek cisnienia)
  Waga/2(Odplyw chmielu) -> Odplyw chmielu/1
  Oproznianie/1 -> Waga/2(Oproznianie)
  Zalaczenie pompy/1 -> Zasilacz hydrauliczny/1(Zalaczenie pompy)
  F551/1 -> Waga/3(Uszkodzenie oprozniania)
  F532/1 -> Zasilacz hydrauliczny/4(Uszkodzenie silnika)
  Sterowanie rusztem/1 -> Sterownik rusztu/2(Nastawa)
  F511/1 -> Zawor doplywu chmielu/2(Dlawienie)
  F512/1 -> Zawor doplywu chmielu/3(Przeciek)
  F513/1 -> Zawor doplywu chmielu/4(Wyciek)
  F514/1 -> Zawor doplywu chmielu/5(Brak)
  Doplyw zasobnika/1 -> Zawor doplywu chmielu/1(Sterowanie)
  Sensor max/1 -> PozycjaDisc/1
  Pozycja sensora max/1 -> Sensor max/2
  Waga/3(Poz dol) -> Waga poz dol/1
  Waga/4(Poz gora) -> Waga poz gora/1
  F541/1 -> Silownik hydrauliczny/2(Uszkodzenie)

== system BrowarModel/System dozowania chmielu/WT505 ==
  note: Przetwornik pomiarowy
  In : Inport
  F_gain : Gain  Gain=0
  F_offset : Constant  Value=0
  GUIMon : Gain
  Kompensacja : Constant  Value=Kompensacja
  Product : Product  RndMeth=Zero
  Quantizer : Quantizer  QuantizationInterval=0.02
  Saturation : Saturate  UpperLimit=100  LowerLimit=0
  Skalowanie (0-100%) : Gain  Gain=100/SrcZakres
  Sum{,1..3} (4 alike) : Sum  Inputs=|++
  Transfer Fcn : TransferFcn  Denominator=[0.3 1]
  Zaklocenia pomiarowe : Subsystem
  Zakres : Constant  Value=Zakres/100
  Out : Outport
  wires:
  Transfer Fcn/1 -> Saturation/1
  F_offset/1 -> Sum3/2
  F_gain/1 -> Sum2/2
  Product/1 -> Sum/1
  Zakres/1 -> Product/2
  Kompensacja/1 -> Sum/2
  Sum/1 -> Quantizer/1
  Skalowanie (0-100%)/1 -> Sum1/1
  Zaklocenia pomiarowe/1(Out) -> Sum1/2
  Sum1/1 -> F_gain/1, Sum2/1
  Sum3/1 -> Transfer Fcn/1
  Sum2/1 -> Sum3/1
  In/1 -> Skalowanie (0-100%)/1
  GUIMon/1 -> Out/1
  Saturation/1 -> Product/1
  Quantizer/1 -> GUIMon/1

== system BrowarModel/System dozowania chmielu/XT504 ==
  note: Przetwornik pomiarowy
  In : Inport
  F_gain : Gain  Gain=0
  F_offset : Constant  Value=0
  GUIMon : Gain
  Kompensacja : Constant  Value=Kompensacja
  Product : Product  RndMeth=Zero
  Saturation : Saturate  UpperLimit=100  LowerLimit=0
  Skalowanie (0-100%) : Gain  Gain=100/SrcZakres
  Sum{,1..3} (4 alike) : Sum  Inputs=|++
  Transfer Fcn : TransferFcn  Denominator=[0.3 1]
  Zaklocenia pomiarowe : Subsystem
  Zakres : Constant  Value=Zakres/100
  Out : Outport
  wires:
  Transfer Fcn/1 -> Saturation/1
  F_offset/1 -> Sum3/2
  F_gain/1 -> Sum2/2
  Product/1 -> Sum/1
  Zakres/1 -> Product/2
  Kompensacja/1 -> Sum/2
  Sum/1 -> GUIMon/1
  Skalowanie (0-100%)/1 -> Sum1/1
  Zaklocenia pomiarowe/1(Out) -> Sum1/2
  Sum1/1 -> F_gain/1, Sum2/1
  Sum3/1 -> Transfer Fcn/1
  Sum2/1 -> Sum3/1
  In/1 -> Skalowanie (0-100%)/1
  GUIMon/1 -> Out/1
  Saturation/1 -> Product/1

== system BrowarModel/System dozowania chmielu/XT504C ==
  note: Przetwornik pomiarowy
  In : Inport
  FT : Constant  Value=0
  FT_value : Constant  Value=0
  GUIMon : Gain
  Switch : Switch  Threshold=0.5  SaturateOnIntegerOverflow=off  InputSameDT=off
  Out : Outport
  wires:
  In/1 -> Switch/3
  GUIMon/1 -> Out/1
  FT/1 -> Switch/2
  Switch/1 -> GUIMon/1
  FT_value/1 -> Switch/1

== system BrowarModel/System dozowania chmielu/XT506H ==
  note: Przetwornik pomiarowy
  In : Inport
  FT : Constant  Value=0
  FT_value : Constant  Value=0
  GUIMon : Gain
  Switch : Switch  Threshold=0.5  SaturateOnIntegerOverflow=off  InputSameDT=off
  Out : Outport
  wires:
  FT_value/1 -> Switch/1
  Switch/1 -> GUIMon/1
  FT/1 -> Switch/2
  GUIMon/1 -> Out/1
  In/1 -> Switch/3

== system BrowarModel/System dozowania chmielu/XT506L ==
  note: Przetwornik pomiarowy
  In : Inport
  FT : Constant  Value=0
  FT_value : Constant  Value=0
  GUIMon : Gain
  Switch : Switch  Threshold=0.5  SaturateOnIntegerOverflow=off  InputSameDT=off
  Out : Outport
  wires:
  In/1 -> Switch/3
  GUIMon/1 -> Out/1
  FT/1 -> Switch/2
  Switch/1 -> GUIMon/1
  FT_value/1 -> Switch/1

== system BrowarModel/System dozowania chmielu/XV504 ==
  note: Sterowanie
  GUIMon : Gain
  Lokalne : Constant  Value=0
  Wybor : Switch  Threshold=0.5  SaturateOnIntegerOverflow=off  InputSameDT=off
  Out : Outport
  wires:
  GUIMon/1 -> Out/1
  Wybor/1 -> GUIMon/1
  [TrybSter] -> Wybor/2
  [XV504] -> Wybor/1
  Lokalne/1 -> Wybor/3

== system BrowarModel/System dozowania chmielu/XV506 ==
  note: Sterowanie
  GUIMon : Gain
  Lokalne : Constant
  Wybor : Switch  Threshold=0.5  SaturateOnIntegerOverflow=off  InputSameDT=off
  Out : Outport
  wires:
  Lokalne/1 -> Wybor/3
  [XV506] -> Wybor/1
  [TrybSter] -> Wybor/2
  Wybor/1 -> GUIMon/1
  GUIMon/1 -> Out/1

== system BrowarModel/System dozowania drozdzy/LT802H ==
  note: Przetwornik pomiarowy
  In : Inport
  FT : Constant  Value=0
  FT_value : Constant  Value=0
  GUIMon : Gain
  Switch : Switch  Threshold=0.5  SaturateOnIntegerOverflow=off  InputSameDT=off
  Out : Outport
  wires:
  In/1 -> Switch/3
  GUIMon/1 -> Out/1
  FT/1 -> Switch/2
  Switch/1 -> GUIMon/1
  FT_value/1 -> Switch/1

== system BrowarModel/System dozowania drozdzy/LT802L ==
  note: Przetwornik pomiarowy
  In : Inport
  FT : Constant  Value=0
  FT_value : Constant  Value=0
  GUIMon : Gain
  Switch : Switch  Threshold=0.5  SaturateOnIntegerOverflow=off  InputSameDT=off
  Out : Outport
  wires:
  FT_value/1 -> Switch/1
  Switch/1 -> GUIMon/1
  FT/1 -> Switch/2
  GUIMon/1 -> Out/1
  In/1 -> Switch/3

== system BrowarModel/System dozowania drozdzy/LV801 ==
  note: Sterowanie
  GUIMon : Gain
  Lokalne : Constant  Value=0
  Wybor : Switch  Threshold=0.5  SaturateOnIntegerOverflow=off  InputSameDT=off
  Out : Outport
  wires:
  GUIMon/1 -> Out/1
  Wybor/1 -> GUIMon/1
  [TrybSter] -> Wybor/2
  [LV801] -> Wybor/1
  Lokalne/1 -> Wybor/3

== system BrowarModel/System dozowania drozdzy/PT803 ==
  note: Przetwornik pomiarowy
  In : Inport
  F_gain : Gain  Gain=0
  F_offset : Constant  Value=0
  GUIMon : Gain
  Kompensacja : Constant  Value=Kompensacja
  Product : Product  RndMeth=Zero
  Saturation : Saturate  UpperLimit=100  LowerLimit=0
  Skalowanie (0-100%) : Gain  Gain=100/SrcZakres
  Sum{,1..3} (4 alike) : Sum  Inputs=|++
  Transfer Fcn : TransferFcn  Denominator=[0.3 1]
  Zaklocenia pomiarowe : Subsystem
  Zakres : Constant  Value=Zakres/100
  Out : Outport
  wires:
  Saturation/1 -> Product/1
  GUIMon/1 -> Out/1
  In/1 -> Skalowanie (0-100%)/1
  Sum2/1 -> Sum3/1
  Sum3/1 -> Transfer Fcn/1
  Sum1/1 -> Sum2/1, F_gain/1
  Zaklocenia pomiarowe/1(Out) -> Sum1/2
  Skalowanie (0-100%)/1 -> Sum1/1
  Sum/1 -> GUIMon/1
  Kompensacja/1 -> Sum/2
  Zakres/1 -> Product/2
  Product/1 -> Sum/1
  F_gain/1 -> Sum2/2
  F_offset/1 -> Sum3/2
  Transfer Fcn/1 -> Saturation/1

== system BrowarModel/System dozowania drozdzy/PV803 ==
  note: Sterowanie
  GUIMon : Gain
  Lokalne : Constant  Value=0
  Wybor : Switch  Threshold=0.5  SaturateOnIntegerOverflow=off  InputSameDT=off
  Out : Outport
  wires:
  Lokalne/1 -> Wybor/3
  [PV803] -> Wybor/1
  [TrybSter] -> Wybor/2
  Wybor/1 -> GUIMon/1
  GUIMon/1 -> Out/1

== system BrowarModel/System dozowania drozdzy/System dozowania drozdzy ==
  note: System dozowania drozdzy
  Doplyw zasobnika : Inport
  Zalaczenie pompy : Inport  Port=2
  Sterowanie rusztem : Inport  Port=3
  Oproznianie : Inport  Port=4
  F{811..814,821,831..832,841,851} (9 alike) : Constant  Value=0
  Pozycja sensora max : Constant  Value=0.1*0.1
  Ruszt dozujacy : Subsystem
  Sensor max : RelationalOperator  InputSameDT=off
  Silownik hydrauliczny : Subsystem
  Sterownik rusztu : Subsystem
  Waga : Subsystem
  Zasilacz hydrauliczny : Subsystem
  Zasobnik : Subsystem
  Zawor doplywu drozdzy : Subsystem  mask{Fmax=0.05}
      mask prompts: Fmax "Przeplyw maksymalny [m3/s]"
  Zawor trojdrozny : Subsystem
  Poziom wysoki zasobnika : Outport
  Poziom niski zasobnika : Outport  Port=2
  Cisnienie pompy : Outport  Port=3
  Masa : Outport  Port=4
  Odplyw drozdzy : Outport  Port=5
  Pozycja : Outport  Port=6
  PozycjaDisc : Outport  Port=7
  Waga poz gora : Outport  Port=8
  Waga poz dol : Outport  Port=9
  wires:
  Sterowanie rusztem/1 -> Sterownik rusztu/2(Nastawa)
  F832/1 -> Zasilacz hydrauliczny/4(Uszkodzenie silnika)
  F851/1 -> Waga/3(Uszkodzenie oprozniania)
  Zalaczenie pompy/1 -> Zasilacz hydrauliczny/1(Zalaczenie pompy)
  Oproznianie/1 -> Waga/2(Oproznianie)
  Waga/2(Odplyw chmielu) -> Odplyw drozdzy/1
  F831/1 -> Zasilacz hydrauliczny/3(Spadek cisnienia)
  Zasilacz hydrauliczny/2(Cisnienie zasilania) -> Cisnienie pompy/1
  Doplyw zasobnika/1 -> Zawor doplywu drozdzy/1(Sterowanie)
  Zawor doplywu drozdzy/1(Przeplyw) -> Zasobnik/1(Doplyw)
  F821/1 -> Zasobnik/3(Wyciek)
  Zasobnik/3(Poziom LO) -> Poziom niski zasobnika/1
  Zasobnik/2(Poziom HI) -> Poziom wysoki zasobnika/1
  Zasobnik/1(Poziom) -> Ruszt dozujacy/2(Poziom_w_zbiorniku)
  Waga/1(Masa) -> Masa/1  "kg"
  Sterownik rusztu/1(Sterowanie zaworem) -> Zawor trojdrozny/1(Sterowanie rusztem)
  Zasilacz hydrauliczny/1(Max przeplyw zasilanie) -> Zawor trojdrozny/2(Przeplyw zasilanie)
  Zawor trojdrozny/1(Przeplyw sterowanie) -> Silownik hydrauliczny/1(Przeplyw zasilanie)
  Silownik hydrauliczny/2(Przeplyw pobor) -> Zasilacz hydrauliczny/2(Przeplyw_pobor)
  Silownik hydrauliczny/1(Pozycja) -> Ruszt dozujacy/1(Pozycja), Sensor max/1, Pozycja/1, Sterownik rusztu/1(Pozycja rusztu)
  Ruszt dozujacy/1(Przeplyw) -> Waga/1(Doplyw), Zasobnik/2(Odplyw)
  F811/1 -> Zawor doplywu drozdzy/2(Dlawienie)
  F812/1 -> Zawor doplywu drozdzy/3(Przeciek)
  F813/1 -> Zawor doplywu drozdzy/4(Wyciek)
  F814/1 -> Zawor doplywu drozdzy/5(Brak)
  Waga/3(Poz dol) -> Waga poz dol/1
  Waga/4(Poz gora) -> Waga poz gora/1
  F841/1 -> Silownik hydrauliczny/2(Uszkodzenie)
  Sensor max/1 -> PozycjaDisc/1
  Pozycja sensora max/1 -> Sensor max/2

== system BrowarModel/System dozowania drozdzy/WT805 ==
  note: Przetwornik pomiarowy
  In : Inport
  F_gain : Gain  Gain=0
  F_offset : Constant  Value=0
  GUIMon : Gain
  Kompensacja : Constant  Value=Kompensacja
  Product : Product  RndMeth=Zero
  Quantizer : Quantizer  QuantizationInterval=0.02
  Saturation : Saturate  UpperLimit=100  LowerLimit=0
  Skalowanie (0-100%) : Gain  Gain=100/SrcZakres
  Sum{,1..3} (4 alike) : Sum  Inputs=|++
  Transfer Fcn : TransferFcn  Denominator=[0.3 1]
  Zaklocenia pomiarowe : Subsystem
  Zakres : Constant  Value=Zakres/100
  Out : Outport
  wires:
  Transfer Fcn/1 -> Saturation/1
  F_offset/1 -> Sum3/2
  F_gain/1 -> Sum2/2
  Product/1 -> Sum/1
  Zakres/1 -> Product/2
  Kompensacja/1 -> Sum/2
  Sum/1 -> Quantizer/1
  Skalowanie (0-100%)/1 -> Sum1/1
  Zaklocenia pomiarowe/1(Out) -> Sum1/2
  Sum1/1 -> F_gain/1, Sum2/1
  Sum3/1 -> Transfer Fcn/1
  Sum2/1 -> Sum3/1
  In/1 -> Skalowanie (0-100%)/1
  GUIMon/1 -> Out/1
  Saturation/1 -> Product/1
  Quantizer/1 -> GUIMon/1

== system BrowarModel/System dozowania drozdzy/XT804 ==
  note: Przetwornik pomiarowy
  In : Inport
  F_gain : Gain  Gain=0
  F_offset : Constant  Value=0
  GUIMon : Gain
  Kompensacja : Constant  Value=Kompensacja
  Product : Product  RndMeth=Zero
  Saturation : Saturate  UpperLimit=100  LowerLimit=0
  Skalowanie (0-100%) : Gain  Gain=100/SrcZakres
  Sum{,1..3} (4 alike) : Sum  Inputs=|++
  Transfer Fcn : TransferFcn  Denominator=[0.3 1]
  Zaklocenia pomiarowe : Subsystem
  Zakres : Constant  Value=Zakres/100
  Out : Outport
  wires:
  Transfer Fcn/1 -> Saturation/1
  F_offset/1 -> Sum3/2
  F_gain/1 -> Sum2/2
  Product/1 -> Sum/1
  Zakres/1 -> Product/2
  Kompensacja/1 -> Sum/2
  Sum/1 -> GUIMon/1
  Skalowanie (0-100%)/1 -> Sum1/1
  Zaklocenia pomiarowe/1(Out) -> Sum1/2
  Sum1/1 -> F_gain/1, Sum2/1
  Sum3/1 -> Transfer Fcn/1
  Sum2/1 -> Sum3/1
  In/1 -> Skalowanie (0-100%)/1
  GUIMon/1 -> Out/1
  Saturation/1 -> Product/1

== system BrowarModel/System dozowania drozdzy/XT804C ==
  note: Przetwornik pomiarowy
  In : Inport
  FT : Constant  Value=0
  FT_value : Constant  Value=0
  GUIMon : Gain
  Switch : Switch  Threshold=0.5  SaturateOnIntegerOverflow=off  InputSameDT=off
  Out : Outport
  wires:
  In/1 -> Switch/3
  GUIMon/1 -> Out/1
  FT/1 -> Switch/2
  Switch/1 -> GUIMon/1
  FT_value/1 -> Switch/1
